simulink model "model_from_metod"  (R2016a)
settings: Solver=VariableStepAuto  StartTime=0.0  StopTime=2  RelTol=1e-3
values from neighbouring files (symbols this model uses):
  A = [0 0 1 ... (first row only)    [start.m]
  B = [0 ... (first row only)    [start.m]
  D = 0.07    [params.m]    (also in start.m = zeros(3, 1))
  K = lqr(s1, QQ, RR)    [control.m]    (also in controlEV3.m = lqrd(s1.A,s1.B, QQ, RR, Ts); control_A.m = QQ*Inv(Y)*; control_P.m = (inv(AA)*BB)')
  Psi0 = 0.15    [params.m]
  Psi_d0 = 0    [params.m]
  R = 0.0275    [params.m]
  Theta_d0 = 0    [params.m]
libraries: vrlib x4, simulink_extras x3
settings Model: Creator=Vlad  LastModifiedBy=Vlad
settings DataIOCC: TimeSaveName=m_tout

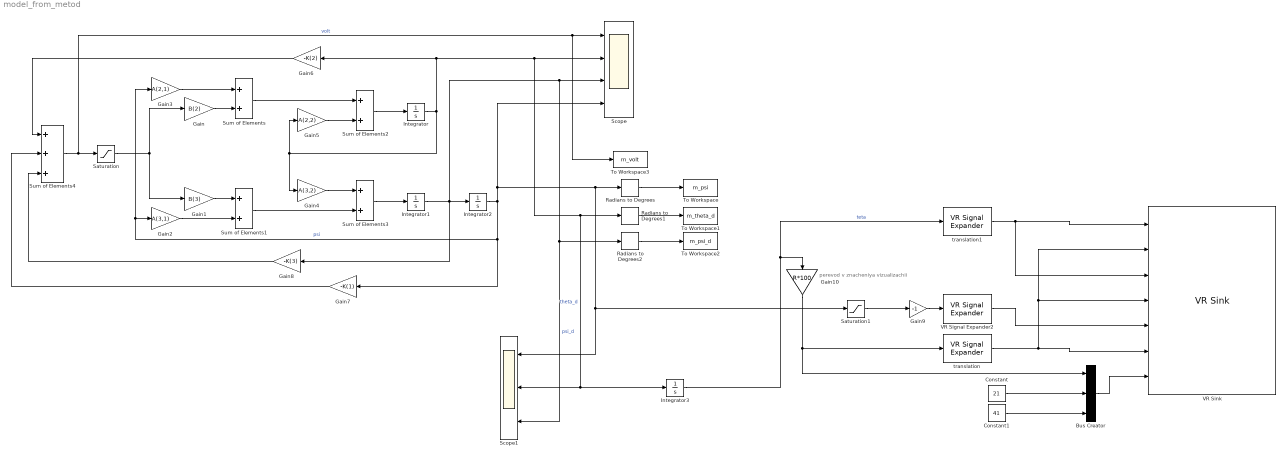
== system model_from_metod ==
  note: perevod v znacheniya vizualizachii
  Bus Creator : BusCreator  Inputs=3
  Constant : Constant  Value=21
  Constant1 : Constant  Value=41
  Gain : Gain  Gain=B(2)
  Gain1 : Gain  Gain=B(3)
  Gain10 : Gain  Gain=R*100
  Gain2 : Gain  Gain=A(3,1)
  Gain3 : Gain  Gain=A(2,1)
  Gain4 : Gain  Gain=A(3,2)
  Gain5 : Gain  Gain=A(2,2)
  Gain6 : Gain  Gain=-K(2)
  Gain7 : Gain  Gain=-K(1)
  Gain8 : Gain  Gain=-K(3)
  Gain9 : Gain  Gain=-1
  Integrator : Integrator  InitialCondition=Theta_d0
  Integrator1 : Integrator  InitialCondition=Psi_d0
  Integrator2 : Integrator  InitialCondition=Psi0
  Integrator3 : Integrator
  Radians to Degrees : simulink_extras/Transformations/Radians to Degrees
  Radians to Degrees1 : simulink_extras/Transformations/Radians to Degrees
  Radians to Degrees2 : simulink_extras/Transformations/Radians to Degrees
  Saturation : Saturate  UpperLimit=100  LowerLimit=-100
  Saturation1 : Saturate  UpperLimit=pi/2  LowerLimit=-pi/2
  Scope : Scope  NumInputPorts=4
  Scope1 : Scope  NumInputPorts=3
  Sum of Elements{,1..3} (4 alike) : Sum  Inputs=2
  Sum of Elements4 : Sum  Inputs=3
  To Workspace : ToWorkspace  VariableName=m_psi  SampleTime=-1
  To Workspace1 : ToWorkspace  VariableName=m_theta_d  SampleTime=-1
  To Workspace2 : ToWorkspace  VariableName=m_psi_d  SampleTime=-1
  To Workspace3 : ToWorkspace  VariableName=m_volt  SampleTime=-1
  VR Signal Expander2 : vrlib/VR Signal Expander  outwidth=4  outidx=[4]
  VR Sink : vrlib/VR Sink  InstantiateOnLoad=on  SampleTime=0.005  ViewEnable=on  RemoteChange=off  RemoteView=off  FieldsWritten=weel1.rotation.4.1.1.double#weel1.translation.3.1.1.double#weel2.rotation.4.1.1.double#weel2.translation.3.1.1.double#Box.rotation.4.1.1.double#Box.translation.3.1.1.double#first.position.3.1.1.double  WorldFileName=D:\VPD\segway.WRL  AutoView=off  VideoDimensions=[]  AllowVariableSize=off
  translation : vrlib/VR Signal Expander  outwidth=3  outidx=[1]
  translation1 : vrlib/VR Signal Expander  outwidth=4  outidx=[1]
  wires:
  Saturation/1 -> Gain1/1, Gain/1
  Gain/1 -> Sum of Elements/2
  Gain1/1 -> Sum of Elements1/1
  Gain2/1 -> Sum of Elements1/2
  Gain3/1 -> Sum of Elements/1
  Sum of Elements/1 -> Sum of Elements2/1
  Sum of Elements1/1 -> Sum of Elements3/2
  Gain5/1 -> Sum of Elements2/2
  Gain4/1 -> Sum of Elements3/1
  Sum of Elements2/1 -> Integrator/1
  Sum of Elements3/1 -> Integrator1/1
  Integrator/1 -> Gain6/1, Integrator3/1, Scope1/2, Radians to Degrees1/1, Scope/2, Gain4/1, Gain5/1  "theta_d"
  Integrator1/1 -> Scope1/3, Radians to Degrees2/1, Scope/3, Gain8/1, Integrator2/1  "psi_d"
  Sum of Elements4/1 -> To Workspace3/1, Scope/1, Saturation/1  "volt"
  Gain6/1 -> Sum of Elements4/1
  Gain7/1 -> Sum of Elements4/2
  Gain8/1 -> Sum of Elements4/3
  Radians to Degrees/1 -> To Workspace/1
  Radians to Degrees2/1 -> To Workspace2/1
  Radians to Degrees1/1 -> To Workspace1/1
  Integrator2/1 -> Scope/4, Saturation1/1, Scope1/1, Radians to Degrees/1, Gain7/1, Gain2/1, Gain3/1  "psi"
  Integrator3/1 -> translation1/1, Gain10/1  "teta"
  translation/1 -> VR Sink/2, VR Sink/4, VR Sink/6
  VR Signal Expander2/1 -> VR Sink/5
  translation1/1 -> VR Sink/3, VR Sink/1
  Gain9/1 -> VR Signal Expander2/1
  Bus Creator/1 -> VR Sink/7
  Constant/1 -> Bus Creator/2
  Constant1/1 -> Bus Creator/3
  Gain10/1 -> Bus Creator/1, translation/1
  Saturation1/1 -> Gain9/1
